simulink model "sigmadelta2"  (Simulink 7.4)
settings: Solver=ode45  StartTime=0.0  StopTime=100.0  RelTol=1e-3
settings Model: Creator=Tibor  LastModifiedBy=Tibor

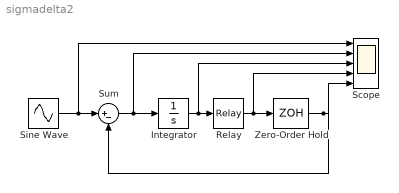
== system sigmadelta2 ==
  Integrator : Integrator
  Relay : Relay  OnSwitchValue=0  OffSwitchValue=0  OffOutputValue=-1  OutDataType=fixdt(1, 16)  OutScaling=2^0
  Scope : Scope  NumInputPorts=5
      settings: YMin=-5~-5~-5~-5~-5  YMax=5~5~5~5~5  SampleInput=on
  Sine Wave : Sin  Amplitude=1  Bias=0  Frequency=0.05  Phase=0  Samples=10  SampleTime=0  Offset=0
  Sum : Sum  Inputs=|+-  OutDataType=fixdt(1, 16)  OutScaling=2^0
  Zero-Order Hold : ZeroOrderHold
  wires:
  Sum/1 -> Integrator/1, Scope/2
  Integrator/1 -> Relay/1, Scope/3
  Zero-Order Hold/1 -> Scope/5, Sum/2
  Relay/1 -> Zero-Order Hold/1, Scope/4
  Sine Wave/1 -> Sum/1, Scope/1
